simulink model "test_exponential_adaptive_smoother"  (R2025b)
settings: Solver=FixedStepAuto  StartTime=0.0  StopTime=0.2  RelTol=1e-3
libraries: arsenal x1
settings Model: Creator=mfussi  LastModifiedBy=mfussi
settings OptimizationCC: DefaultParameterBehavior=Inlined  UseDivisionForNetSlopeComputation=on  GainParamInheritBuiltInType=on  UseFloatMulNetSlope=on  InlineInvariantSignals=on  PassReuseOutputArgsAs=Individual arguments  RollThreshold=2.0  ZeroExternalMemoryAtStartup=off  ZeroInternalMemoryAtStartup=off  NoFixptDivByZeroProtection=on  EfficientFloat2IntCast=on  LifeSpan=1  OptimizeBlockOrder=speed  DifferentSizesBufferReuse=on  EfficientTunableParamExpr=on
settings DebuggingCC: ParameterTunabilityLossMsg=error
settings HardwareCC: ProdBitPerPointer=32.0  ProdBitPerSizeT=32.0  ProdBitPerPtrDiffT=32.0  ProdLargestAtomicInteger=Long  ProdLargestAtomicFloat=Double  ProdWordSize=32.0  ProdLongLongMode=on  ProdHWDeviceType=ARM Compatible->ARM Cortex-M
settings SFSimCC: MATLABDynamicMemAlloc=off
settings RTWCC: SystemTargetFile=ert.tlc  GenCodeOnly=on  TemplateMakefile=ert_default_tmf  TargetLang=C++  Description=Embedded Coder
settings CodeAppCC: ForceParamTrailComments=on  IgnoreCustomStorageClasses=off  OperatorAnnotations=on  SimulinkDataObjDesc=on  SFDataObjDesc=on  CustomSymbolStrGlobalVar=rt$N$M  CustomSymbolStrType=$N$M  CustomSymbolStrFcn=$N$M$F  CustomSymbolStrMacro=$N$M  InsertBlockDesc=on
settings ERTTargetCC: RootIOFormat=Structure reference  ERTCustomFileTemplate=example_file_process.tlc  ERTFilePackagingFormat=CompactWithDataFile  TargetLangStandard=C++11 (ISO)  GenerateSampleERTMain=on  IncludeMdlTerminateFcn=off  CombineSignalStateStructs=on  SupportAbsoluteTime=off  CodeInterfacePackaging=C++ class  SubcomponentCodeInterfacePackaging=C++ class  SupportComplex=off  SupportContinuousTime=on

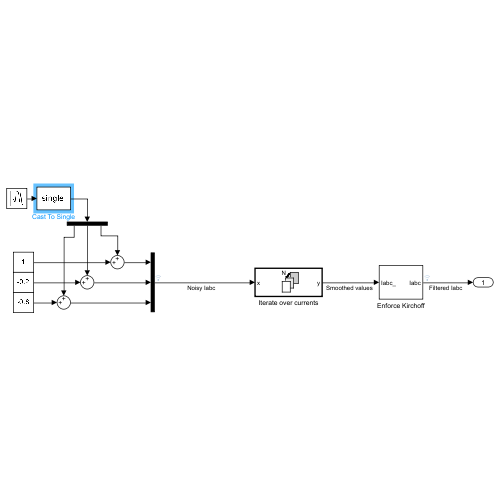
[thumbnail: Simulink's stored preview of the top-level diagram]
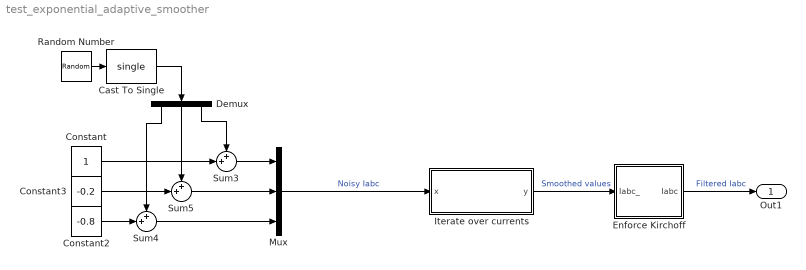
== system test_exponential_adaptive_smoother ==
  Cast To Single : DataTypeConversion  OutDataTypeStr=single  SaturateOnIntegerOverflow=off  RndMeth=Floor
  Constant : Constant  OutDataTypeStr=single
  Constant2 : Constant  Value=-0.8  OutDataTypeStr=single
  Constant3 : Constant  Value=-0.2  OutDataTypeStr=single
  Demux : Demux  Outputs=3
  Enforce Kirchoff : Subsystem
  Iterate over currents : Subsystem  TreatAsAtomicUnit=on
  Mux : Mux  Inputs=3
  Random Number : RandomNumber  Variance=0.02  Seed=[0, 1, 2]  SampleTime=45e-6
  Sum3 : Sum  Inputs=++|
  Sum4 : Sum  Inputs=++|
  Sum5 : Sum  Inputs=++|
  Out1 : Outport
  wires:
  Sum3/1 -> Mux/1
  Sum4/1 -> Mux/3
  Sum5/1 -> Mux/2
  Constant/1 -> Sum3/2
  Constant2/1 -> Sum4/2
  Constant3/1 -> Sum5/2
  Random Number/1 -> Cast To Single/1
  Demux/3 -> Sum3/1
  Demux/2 -> Sum5/1
  Demux/1 -> Sum4/1
  Cast To Single/1 -> Demux/1
  Mux/1 -> Iterate over currents/1(x)  "Noisy Iabc"
  Iterate over currents/1(y) -> Enforce Kirchoff/1(Iabc_)  "Smoothed values"
  Enforce Kirchoff/1(Iabc) -> Out1/1  "Filtered Iabc"

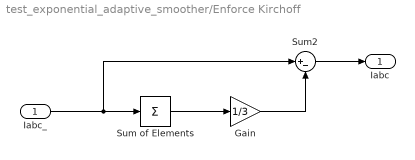
== system test_exponential_adaptive_smoother/Enforce Kirchoff ==
  Iabc_ : Inport
  Gain : Gain  Gain=1/3
  Sum of Elements : Sum  Inputs=+
  Sum2 : Sum  Inputs=|+-
  Iabc : Outport
  wires:
  Gain/1 -> Sum2/2
  Iabc_/1 -> Sum2/1, Sum of Elements/1
  Sum of Elements/1 -> Gain/1
  Sum2/1 -> Iabc/1

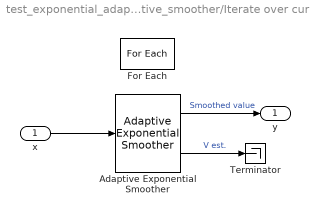
== system test_exponential_adaptive_smoother/Iterate over currents ==
  x : Inport  Partition=on  PartitionDimension=1  PartitionWidth=1  PartitionOffset=0
  Adaptive Exponential Smoother : arsenal/Filters/Adaptive Exponential Smoother  eta=0.003  m=0.99  V0=(1e-3)^2
  For Each : ForEach  DisableCoverage=on
  Terminator : Terminator
  y : Outport  ConcatenationDimension=1
  wires:
  Adaptive Exponential Smoother/1 -> y/1  "Smoothed value"
  x/1 -> Adaptive Exponential Smoother/1
  Adaptive Exponential Smoother/2 -> Terminator/1  "V est."
